simulink model "first"  (Simulink 8.8)
settings: Solver=FixedStepDiscrete  StartTime=0  StopTime=100  RelTol=1e-3  EnableMultiTasking=on
undefined symbols (not defined in the file or in its folder): DiscIntNeverNeededParam
settings Model: Creator=irina  LastModifiedBy=irina
settings OptimizationCC: ExpressionDepthLimit=2147483647
settings DebuggingCC: SolverPrmCheckMsg=warning

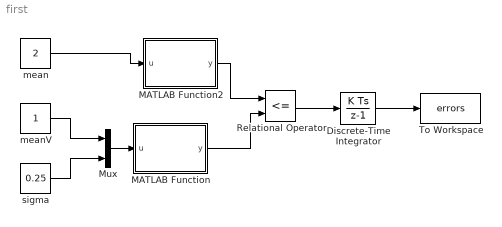
== system first ==
  Discrete-Time Integrator : DiscreteIntegrator  ICPrevOutput=DiscIntNeverNeededParam  ICPrevScaledInput=DiscIntNeverNeededParam
  MATLAB Function : MATLAB Function  TreatAsAtomicUnit=on
  MATLAB Function2 : MATLAB Function  TreatAsAtomicUnit=on
  Mux : Mux  Inputs=2
  Relational Operator : RelationalOperator  Operator=<=  OutDataTypeStr=boolean  RndMeth=Nearest
  To Workspace : ToWorkspace  VariableName=errors  SaveFormat=Structure  SampleTime=-1
  mean : Constant  Value=2
  meanV : Constant
  sigma : Constant  Value=0.25
  wires:
  meanV/1 -> Mux/1
  sigma/1 -> Mux/2
  Mux/1 -> MATLAB Function/1(u)
  MATLAB Function/1(y) -> Relational Operator/2
  Relational Operator/1 -> Discrete-Time Integrator/1
  mean/1 -> MATLAB Function2/1(u)
  MATLAB Function2/1(y) -> Relational Operator/1
  Discrete-Time Integrator/1 -> To Workspace/1

== matlab function MATLAB Function ==
  data: u input double; y output double
function y = fcn(u)
    y = normrnd(u(1),u(2),1,1);
end

== matlab function MATLAB Function2 ==
  data: u input double; y output double
function y = fcn(u)
    y = chi2rnd(u(1),1,1);
end
